simulink model "StateSpaceModelDemo"  (R2022b)
settings: Solver=VariableStepAuto  StartTime=0.0  StopTime=10  FixedStep=0.01  MaxStep=0.05  RelTol=1e-3
values from neighbouring files (symbols this model uses):
  A = [0, 0, 1, 0 ... (first row only)    [demo_state_space_init.m]
  B = [0, 0 ... (first row only)    [demo_state_space_init.m]
  C = [1/2, 1/2, 0, 0 ... (first row only)    [demo_state_space_init.m]
  D = [0, 0 ... (first row only)    [demo_state_space_init.m]
settings Model: Creator=armte  LastModifiedBy=armte

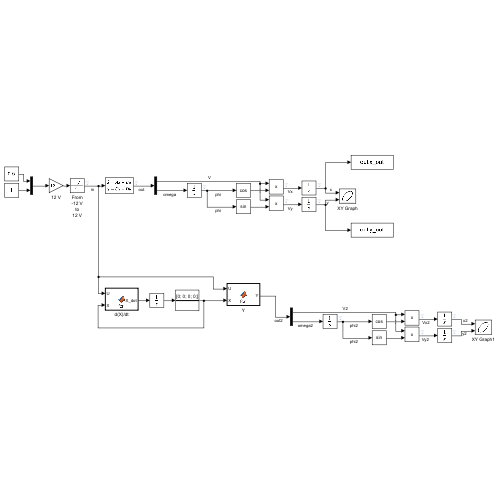
[thumbnail: Simulink's stored preview of the top-level diagram]
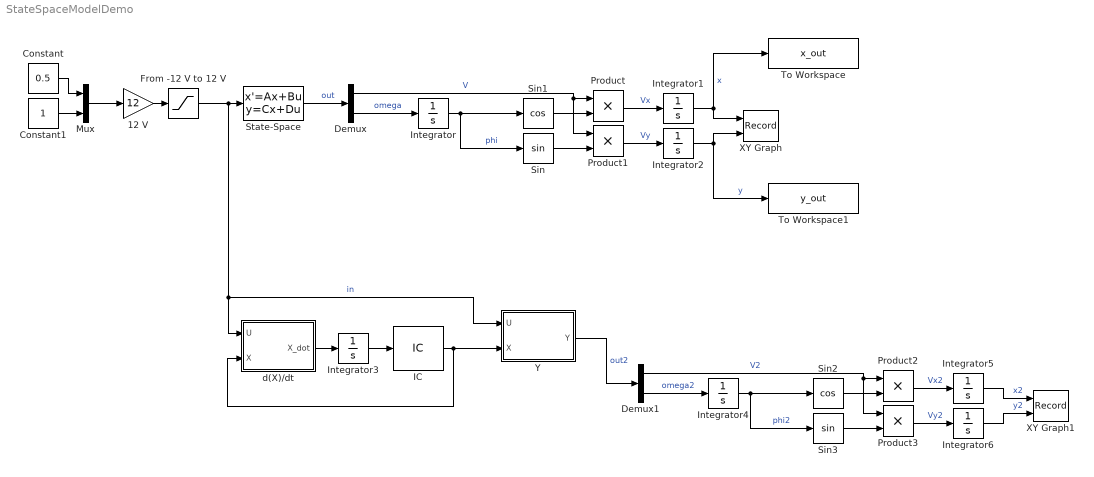
== system StateSpaceModelDemo ==
  12 V : Gain  Gain=12
  Constant : Constant  Value=0.5
  Constant1 : Constant
  Demux : Demux  Outputs=2
  Demux1 : Demux  Outputs=2
  From -12 V to 12 V : Saturate  UpperLimit=12  LowerLimit=-12
  IC : InitialCondition  Value=[0; 0; 0; 0;]
  Integrator{,1..6} (7 alike) : Integrator
  Mux : Mux  Inputs=2
  Product{,1..3} (4 alike) : Product
  Sin : Trigonometry
  Sin1 : Trigonometry  Operator=cos
  Sin2 : Trigonometry  Operator=cos
  Sin3 : Trigonometry
  State-Space : StateSpace  A=A  B=B  C=C  D=D  InitialCondition=0
  To Workspace : ToWorkspace  VariableName=x_out  SampleTime=-1
  To Workspace1 : ToWorkspace  VariableName=y_out  SampleTime=-1
  XY Graph : Record  FileSettingsInternal="{\"entries\":[{\"content\":{\"excelSettings\":{\"content\":{},\"type\":\"Streamout.ExcelSettings\"}},\"type\":\"Streamout.FileSettingStorage\",\"uuid\":\"9bfdd3a5-d0fc-4e1c-b886-b752cda4558f\"}],\"packageUris\":[\"http://schema.mathworks.com/mf0/streamout_blocks/R2020a\"],\"version\":\"1.0\"}"  Layout=[1 1]  SignalsInternal="{\"entries\":[{\"content\":{\"signals\":[{\"content\":{\"blockPath\":[\"StateSpaceModelDemo/XY Graph\"],\"channel\":[],\"dimensions\":[1],\"domain\":\"StateSpaceModelDemo/XY Graph\",\"lineColor\":\"#a2142f\",\"plots\":[1],\"port\":1,\"sid\":[\"\"],\"signalID\":3152,\"signalName\":\"x\"},\"type\":\"RecordBlkView.Signal\",\"uuid\":\"5904ecfd-512f-4a34-870d-ba72ec4437e8\"},{\"content\":{\"blockPath\":[\"StateSpaceModelDemo/XY Graph\"],\"channel\":[],\"dimensions\":[1],\"domain\":\"StateSpaceModelDemo/XY Graph\",\"lineColor\":\"#139fff\",\"plots\":[1],\"port\":2,\"sid\":[\"\"],\"signalID\":3156,\"signalName\":\"y\"},\"type\":\"RecordBlkView.Signal\",\"uuid\":\"dae6ec1b-6a0a-42fd-9e91-b54be02b4f8d\"}]},\"type\":\"RecordBlkView.InputSignals\",\"uuid\":\"35fcb74b-7702-4330-974c-1476f1b396c2\"}],\"packageUris\":[\"http://schema.mathworks.com/mf0/streamout_blocks/R2020a\"],\"version\":\"1.0\"}"  VisualizationBindings="{\"xyplotplugin\":{\"info\":[{\"series\":[{\"bindingParametersList\":[{\"parameter\":\"X-Axis\",\"signalID\":3152,\"signalName\":\"x\"},{\"parameter\":\"Y-Axis\",\"signalID\":3156,\"signalName\":\"y\"}],\"seriesID\":46448}],\"subplotID\":1}]}}"  CompatibilityTag=XY
  XY Graph1 : Record  FileSettingsInternal="{\"entries\":[{\"content\":{\"excelSettings\":{\"content\":{},\"type\":\"Streamout.ExcelSettings\"}},\"type\":\"Streamout.FileSettingStorage\",\"uuid\":\"8dd78601-c387-40cb-a46c-00bc69ac2661\"}],\"packageUris\":[\"http://schema.mathworks.com/mf0/streamout_blocks/R2020a\"],\"version\":\"1.0\"}"  Layout=[1 1]  SignalsInternal="{\"entries\":[{\"content\":{\"signals\":[{\"content\":{\"blockPath\":[\"StateSpaceModelDemo/XY Graph1\"],\"channel\":[],\"dimensions\":[1,1],\"domain\":\"StateSpaceModelDemo/XY Graph1\",\"lineColor\":\"#a2142f\",\"plots\":[1],\"port\":1,\"sid\":[\"\"],\"signalID\":3160,\"signalName\":\"x2\"},\"type\":\"RecordBlkView.Signal\",\"uuid\":\"411b24f0-bd24-4970-86cc-936a57cea44d\"},{\"content\":{\"blockPath\":[\"StateSpaceModelDemo/XY Graph1\"],\"channel\":[],\"dimensions\":[1,1],\"domain\":\"StateSpaceModelDemo/XY Graph1\",\"lineColor\":\"#139fff\",\"plots\":[1],\"port\":2,\"sid\":[\"\"],\"signalID\":3164,\"signalName\":\"y2\"},\"type\":\"RecordBlkView.Signal\",\"uuid\":\"e8ea95b1-6156-4e5a-9633-310ebf80070e\"}]},\"type\":\"RecordBlkView.InputSignals\",\"uuid\":\"4af5ac03-a35e-47a0-90ca-8dfbd49bd5af\"}],\"packageUris\":[\"http://schema.mathworks.com/mf0/streamout_blocks/R2020a\"],\"version\":\"1.0\"}"  VisualizationBindings="{\"xyplotplugin\":{\"info\":[{\"series\":[{\"bindingParametersList\":[{\"parameter\":\"X-Axis\",\"signalID\":3160,\"signalName\":\"x2\"},{\"parameter\":\"Y-Axis\",\"signalID\":3164,\"signalName\":\"y2\"}],\"seriesID\":30010}],\"subplotID\":1}]}}"  CompatibilityTag=XY
  Y : MATLAB Function  TreatAsAtomicUnit=on
  d(X)/dt : MATLAB Function  TreatAsAtomicUnit=on
  wires:
  State-Space/1 -> Demux/1  "out"
  Demux/1 -> Product/1, Product1/1  "V"
  Demux/2 -> Integrator/1  "omega"
  Integrator/1 -> Sin/1, Sin1/1  "phi"
  Sin1/1 -> Product/2
  Sin/1 -> Product1/2
  Product/1 -> Integrator1/1  "Vx"
  Product1/1 -> Integrator2/1  "Vy"
  Integrator1/1 -> XY Graph/1, To Workspace/1  "x"
  Integrator2/1 -> XY Graph/2, To Workspace1/1  "y"
  Constant/1 -> Mux/1
  Constant1/1 -> Mux/2
  12 V/1 -> From -12 V to 12 V/1
  From -12 V to 12 V/1 -> Y/1(U), d(X)/dt/1(U), State-Space/1  "in"
  Mux/1 -> 12 V/1
  d(X)/dt/1(X_dot) -> Integrator3/1
  Integrator3/1 -> IC/1
  IC/1 -> d(X)/dt/2(X), Y/2(X)
  Integrator6/1 -> XY Graph1/2  "y2"
  Integrator5/1 -> XY Graph1/1  "x2"
  Product2/1 -> Integrator5/1  "Vx2"
  Sin2/1 -> Product2/2
  Integrator4/1 -> Sin3/1, Sin2/1  "phi2"
  Demux1/2 -> Integrator4/1  "omega2"
  Demux1/1 -> Product3/1, Product2/1  "V2"
  Y/1(Y) -> Demux1/1  "out2"
  Product3/1 -> Integrator6/1  "Vy2"
  Sin3/1 -> Product3/2

== matlab function StateSpaceModelDemo/d(X)//dt ==
  data: U input; X_dot output; X input
function X_dot = fcn(U, X)

Rwheel = 0.05; % m
Tr = 0.1; % m
Jsum = 0.4; % kg*m^2
R = 10; % Om
L = 650e-6; % H
Km = 0.17;
Komega = 0.17;

A = [0, 0, 1, 0;
     0, 0, 0, 1;
    -Km*Komega/(L*Jsum), 0, -R/L, 0;
    0, -Km*Komega/(L*Jsum), 0, -R/L];

B = [0, 0;
     0, 0;
    Rwheel*Km/(L*Jsum), 0;
    0, Rwheel*Km/(L*Jsum)];

%%
X_dot = A*X + B*U;
end

== matlab function StateSpaceModelDemo/Y ==
  data: U input; Y output; X input
function Y = fcn(U, X)

Rwheel = 0.05; % m
Tr = 0.1; % m
Jsum = 0.4; % kg*m^2
R = 10; % Om
L = 650e-6; % H
Km = 0.17;
Komega = 0.17;

C = [1/2, 1/2, 0, 0;
    -1/Tr, 1/Tr, 0, 0];

D = [0, 0;
     0, 0];

%%
Y = C*X + D*U;
end
